simulink model "bandpass_temp"  (R2013a)
settings: Solver=ode45  StartTime=0.0  StopTime=10.0  RelTol=1e-3
values from neighbouring files (symbols this model uses):
  WM = WM_Sim_config(Time_length,Approx_char_rate,Tx_approx_BW,Carrier_Freq,hopping_approx_frequency,                                       hopping,Frame_len,suppression_filter,supp_filt_order,Eb_N0_dB,'noise',fec,fec_ratio)    [WM_Sim_config_smlnk_standalone.m]
settings Model: Creator=leonardo  LastModifiedBy=leonardo

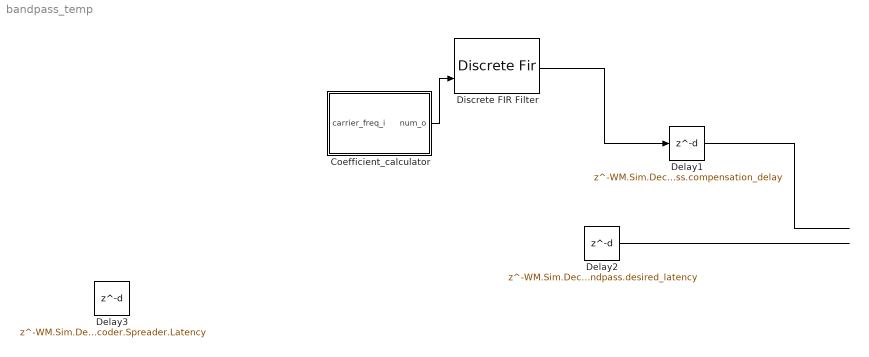
== system bandpass_temp ==
  Coefficient_calculator : Subsystem
  Delay1 : Delay  DelayLength=WM.Sim.Decoder.Bandpass.compensation_delay  InputProcessing=Columns as channels (frame based)
  Delay2 : Delay  DelayLength=WM.Sim.Decoder.Bandpass.desired_latency  InputProcessing=Columns as channels (frame based)
  Delay3 : Delay  DelayLength=WM.Sim.Decoder.Spreader.Latency  InputProcessing=Columns as channels (frame based)
  Discrete FIR Filter : DiscreteFir  CoefSource=Input port  FilterStructure=Direct form transposed  Coefficients=WM.Sim.Decoder.Bandpass.Hd.Numerator  InputProcessing=Columns as channels (frame based)  SampleTime=WM.Sim.SampleTimes.Tchannel
  wires:
  ? -> Delay2/1
  Delay1/1 -> ?
  Delay2/1 -> ?
  Coefficient_calculator/1(num_o) -> Discrete FIR Filter/2
  ? -> Discrete FIR Filter/1
  Discrete FIR Filter/1 -> Delay1/1
  ? -> Coefficient_calculator/1(carrier_freq_i)

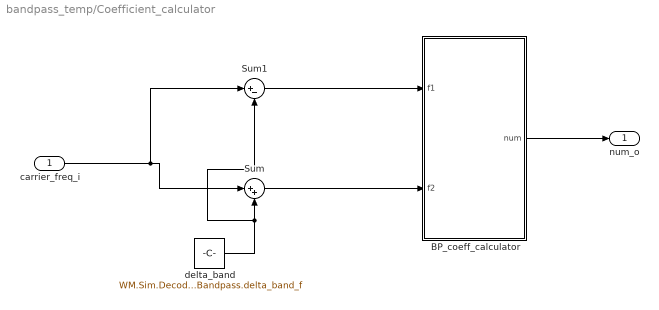
== system bandpass_temp/Coefficient_calculator ==
  carrier_freq_i : Inport
  BP_coeff_calculator : MATLAB Function  TreatAsAtomicUnit=on
  Sum : Sum  Inputs=|++
  Sum1 : Sum  Inputs=|+-
  delta_band : Constant  Value=WM.Sim.Decoder.Bandpass.delta_band_f
  num_o : Outport
  wires:
  BP_coeff_calculator/1(num) -> num_o/1
  Sum1/1 -> BP_coeff_calculator/1(f1)
  delta_band/1 -> Sum1/2, Sum/2
  carrier_freq_i/1 -> Sum1/1, Sum/1
  Sum/1 -> BP_coeff_calculator/2(f2)

== matlab function bandpass_temp/Coefficient_calculator/BP_coeff_calculator ==
  settings: updateMethod=DISCRETE  sampleTime=WM.Sim.SampleTimes.Tchannel
  data: num output; f1 input; f2 input; WM parameter
function num = get_bp_coeffs (f1,f2, WM)

%#codegen
fs = WM.Sim.Fs_audio;

% B=(f2-f1)/fs; % calcola l'ampiezza complessiva della banda normalizzata a fs
%
% Calcola la risposta a 73 coefficienti, simmetrici intorno allo 0
grpdel=WM.Sim.Decoder.Bandpass.grpdel;

filter_length=grpdel*2+1;
h=zeros(1,filter_length);
window=zeros(filter_length,1);
%
w1=2*pi*f1/fs;
w2=2*pi*f2/fs;
for ii=1:grpdel,
h(ii+1+grpdel)=(sin(w2*ii)-sin(w1*ii))/(pi*ii);
h(grpdel+1-ii)=h(ii+1+grpdel);
end
h(grpdel+1)=(w2-w1)/pi;
%
%coefficienti del filtro
window(:,1)=hanning(filter_length);
num=window'.*h;
% norm=sum(hfiltro);
% hfiltro=hfiltro/norm;

% figure
% plot(20*log10(abs(fft(hfiltro))));

% Fc=(f1+f2)/2;
% wc=2*pi*Fc/fs.*(0:length(hfiltro)-1);
% % time = 0:1/fs:length(hfiltro)*1/fs-1/fs;
% num=hfiltro.*exp(wc*1i);

end
